simulink library "Differential_Components"  (R2026a)
settings: Solver=VariableStepAuto
undefined symbols (not defined in the file): Visual, X, Y, Z
libraries: sm_lib x3
Description:
  | Component of Simscape Vehicle Templates Library
  | 
  | Copyright 2018-2026 The MathWorks, Inc.
settings Model: Creator=smiller  LastModifiedBy=smiller

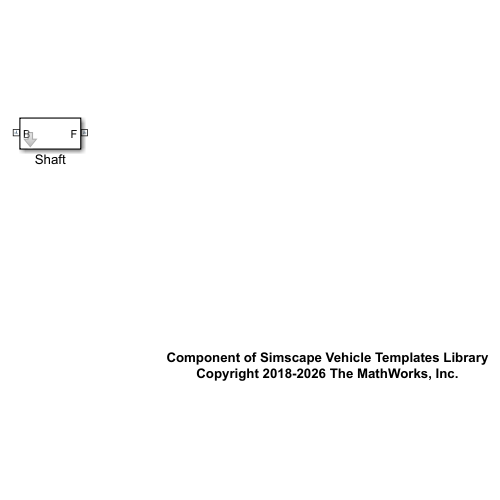
[thumbnail: Simulink's stored preview of the top-level diagram]
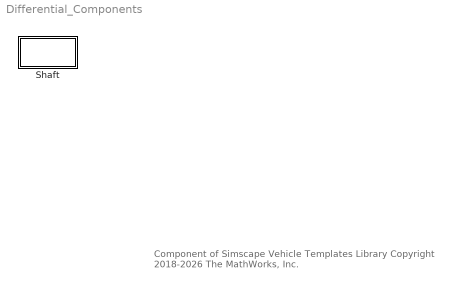
== system Differential_Components ==
  note: Component of Simscape Vehicle Templates Library
      | Copyright 2018-2026 The MathWorks, Inc.
  Shaft : Subsystem  mask(Rigid Shaft){popup_leftRight=Left, shaft_m=3.5, len_shaft=0.4, clr_shaft=Visual.Driveshaft.clr, opc_shaft=Visual.part.opc, rad_shaft=Visual.Driveshaft.rad}
      mask prompts: popup_leftRight "Left/Right"; shaft_m "Shaft Mass (kg)"; len_shaft "Shaft Length (m)"; clr_shaft "Color [RGB]"; opc_shaft "Opacity (0-1)"; rad_shaft "Radius (m)"
      mask help: Models a rigid shaft. Selecting Left or Right will ensure the z-axis points the same way if it is mounted on the left or right side of the vehicle.
      mask init:
      | if(popup_leftRight == 1)
      |     rhs_shaft = 1;
      | elseif(popup_leftRight == 2)
      |     rhs_shaft = -1;
      | end
      mask TypeOptions popup_leftRight: Left | Right
      mask TypeOptions shaft_m: Shaft/Mass
      mask TypeOptions clr_shaft: Shaft/GraphicDiffuseColor
      mask TypeOptions opc_shaft: Shaft/GraphicOpacity
      mask TypeOptions rad_shaft: Shaft/CylinderRadius
      mask DialogControl cont_vis_shaft Prompt: Visualization

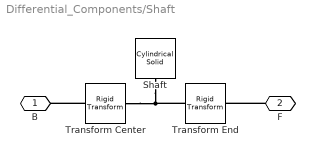
== system Differential_Components/Shaft ==
  Shaft : sm_lib/Body Elements/Cylindrical Solid  CylinderRadius=rad_shaft  CylinderRadiusUnits=m  CylinderLength=len_shaft  CylinderLengthUnits=m  ExportEntireGeometry=off  InertiaType=CalculateFromGeometry  BasedOnType=Mass  Density=1000  DensityUnits=kg/m^3  Mass=shaft_m  MassUnits=kg  CenterOfMass=[0 0 0]  CenterOfMassUnits=m  MomentsOfInertia=[1 1 1]  MomentsOfInertiaUnits=kg*m^2  ProductsOfInertia=[0 0 0]  ProductsOfInertiaUnits=kg*m^2  GraphicType=FromGeometry  MarkerShape=Sphere  MarkerSize=10  GraphicVisPropType=SimpleVisualProperties  GraphicDiffuseColor=clr_shaft  GraphicOpacity=opc_shaft  GraphicSpecularColor=[0.5 0.5 0.5 1.0]  GraphicAmbientColor=[0.15 0.15 0.15 1.0]  GraphicEmissiveColor=[0.0 0.0 0.0 1.0]  GraphicShininess=75  DoExposeReferenceFrame=on  SerializedFrames=<Frames/>
  Transform Center : sm_lib/Frames and Transforms/Rigid Transform  RotationMethod=None  FollAlignAxisA=+X  BaseAlignAxisA=+Y  FollAlignAxisB=+Y  BaseAlignAxisB=+Z  RotationStandardAxis=+Y  RotationAngle=0  RotationAngleUnits=deg  RotationArbitraryAxis=[0 0 1]  RotationSequenceAxes=FollowerAxes  RotationSequence=XYX  RotationSequenceAngles=[0 0 0]  RotationSequenceAnglesUnits=deg  RotationMatrix=[1 0 0; 0 1 0; 0 0 1]  Quaternion=[1 0 0 0]  TranslationMethod=StandardAxis  TranslationCartesianOffset=[0 0 0]  TranslationCartesianOffsetUnits=m  TranslationStandardAxis=-Z  TranslationStandardOffset=len_shaft/2*rhs_shaft  TranslationStandardOffsetUnits=m  TranslationROffset=0  TranslationROffsetUnits=m  TranslationThetaOffset=0  TranslationThetaOffsetUnits=deg  TranslationZOffset=0  TranslationZOffsetUnits=m
  Transform End : sm_lib/Frames and Transforms/Rigid Transform  RotationMethod=None  FollAlignAxisA=+X  BaseAlignAxisA=+Y  FollAlignAxisB=+Y  BaseAlignAxisB=+Z  RotationStandardAxis=+Y  RotationAngle=0  RotationAngleUnits=deg  RotationArbitraryAxis=[0 0 1]  RotationSequenceAxes=FollowerAxes  RotationSequence=XYX  RotationSequenceAngles=[0 0 0]  RotationSequenceAnglesUnits=deg  RotationMatrix=[1 0 0; 0 1 0; 0 0 1]  Quaternion=[1 0 0 0]  TranslationMethod=StandardAxis  TranslationCartesianOffset=[0 0 0]  TranslationCartesianOffsetUnits=m  TranslationStandardAxis=-Z  TranslationStandardOffset=len_shaft/2*rhs_shaft  TranslationStandardOffsetUnits=m  TranslationROffset=0  TranslationROffsetUnits=m  TranslationThetaOffset=0  TranslationThetaOffsetUnits=deg  TranslationZOffset=0  TranslationZOffsetUnits=m
  B : PMIOPort  Side=Left
  F : PMIOPort  Port=2  Side=Right
  connections:
  F/RConn1 -- Transform End/RConn1
  Transform Center/LConn1 -- B/RConn1
  Shaft/RConn1 -- Transform Center/RConn1 -- Transform End/LConn1
